simulink model "PacemakerCells"  (Simulink 7.1)
settings: Solver=ode45  StartTime=0.0  StopTime=0.5  RelTol=1e-3
libraries: NeuroModelerLibrary x11
settings Model: Creator=Bakhshiev  LastModifiedBy=Timba

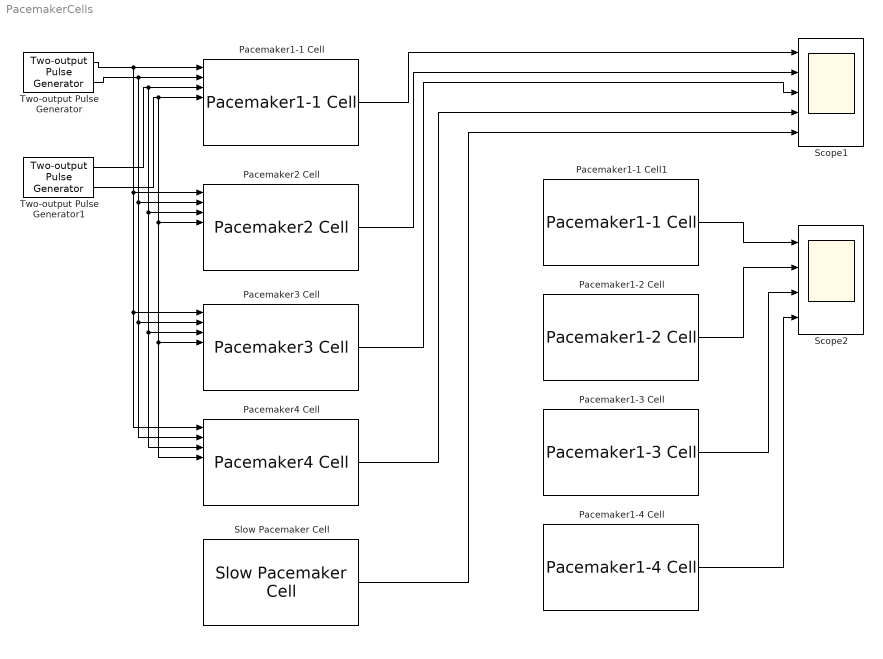
== system PacemakerCells ==
  Pacemaker1-1 Cell : NeuroModelerLibrary/Pacemaker Cells/Pacemaker1-1 Cell  SystemSampleTime=-1
  Pacemaker1-1 Cell1 : NeuroModelerLibrary/Pacemaker Cells/Pacemaker1-1 Cell  SystemSampleTime=-1
  Pacemaker1-2 Cell : NeuroModelerLibrary/Pacemaker Cells/Pacemaker1-2 Cell  SystemSampleTime=-1
  Pacemaker1-3 Cell : NeuroModelerLibrary/Pacemaker Cells/Pacemaker1-3 Cell  SystemSampleTime=-1
  Pacemaker1-4 Cell : NeuroModelerLibrary/Pacemaker Cells/Pacemaker1-4 Cell  SystemSampleTime=-1
  Pacemaker2 Cell : NeuroModelerLibrary/Pacemaker Cells/Pacemaker2 Cell  SystemSampleTime=-1
  Pacemaker3 Cell : NeuroModelerLibrary/Pacemaker Cells/Pacemaker3 Cell  SystemSampleTime=-1
  Pacemaker4 Cell : NeuroModelerLibrary/Pacemaker Cells/Pacemaker4 Cell  SystemSampleTime=-1
  Scope1 : Scope  NumInputPorts=5
      settings: YMin=-0.25~-0.25~-0.25~-0.25~-0.25  YMax=1~1~1~1~1  MaxDataPoints=5000000
  Scope2 : Scope  NumInputPorts=4
      settings: YMin=-0.25~-0.25~-0.25~-0.25  YMax=1~1~1~1  MaxDataPoints=5000000
  Slow Pacemaker Cell : NeuroModelerLibrary/Pacemaker Cells/Slow Pacemaker Cell  SystemSampleTime=-1
  Two-output Pulse Generator : NeuroModelerLibrary/Support/Two-output Pulse Generator  SystemSampleTime=-1  A=1  P1=200  P2=200  PW=1  ST=0.001  OOn1=10.5  OOff1=0.6  OOn2=10.1  OOff2=1.2
  Two-output Pulse Generator1 : NeuroModelerLibrary/Support/Two-output Pulse Generator  SystemSampleTime=-1  A=1  P1=200  P2=200  PW=1  ST=0.001  OOn1=10.5  OOff1=0.6  OOn2=11.1  OOff2=1.2
  wires:
  Two-output Pulse Generator/1 -> Pacemaker3 Cell/1, Pacemaker4 Cell/1, Pacemaker2 Cell/1, Pacemaker1-1 Cell/1
  Two-output Pulse Generator/2 -> Pacemaker3 Cell/2, Pacemaker4 Cell/2, Pacemaker2 Cell/2, Pacemaker1-1 Cell/2
  Two-output Pulse Generator1/2 -> Pacemaker3 Cell/4, Pacemaker4 Cell/4, Pacemaker2 Cell/4, Pacemaker1-1 Cell/4
  Two-output Pulse Generator1/1 -> Pacemaker3 Cell/3, Pacemaker4 Cell/3, Pacemaker2 Cell/3, Pacemaker1-1 Cell/3
  Pacemaker1-1 Cell/2 -> Scope1/1
  Pacemaker2 Cell/2 -> Scope1/2
  Pacemaker3 Cell/2 -> Scope1/3
  Pacemaker4 Cell/2 -> Scope1/4
  Slow Pacemaker Cell/2 -> Scope1/5
  Pacemaker1-1 Cell1/2 -> Scope2/1
  Pacemaker1-2 Cell/2 -> Scope2/2
  Pacemaker1-3 Cell/2 -> Scope2/3
  Pacemaker1-4 Cell/2 -> Scope2/4
